simulink model "Expt2b"  (R2020b)
settings: Solver=VariableStepAuto  StartTime=0.0  StopTime=1.5  RelTol=1e-3
settings Model: Creator=geniu  LastModifiedBy=geniu

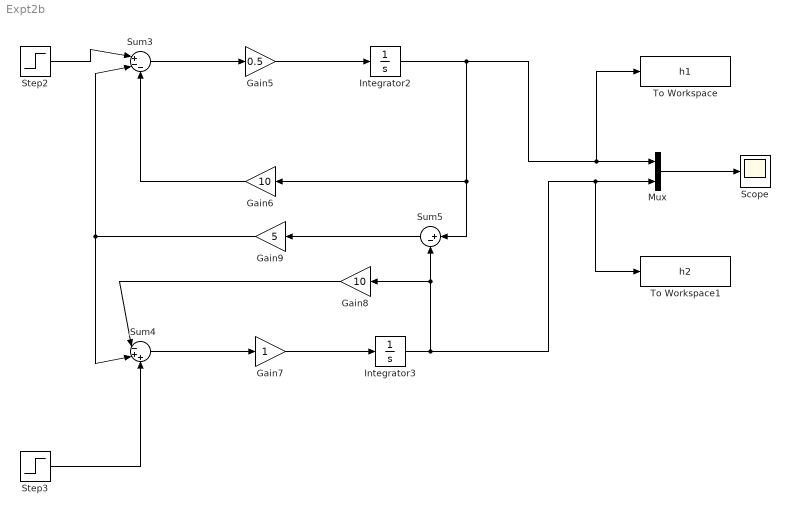
== system Expt2b ==
  Gain5 : Gain  Gain=0.5
  Gain6 : Gain  Gain=10
  Gain7 : Gain
  Gain8 : Gain  Gain=10
  Gain9 : Gain  Gain=5
  Integrator2 : Integrator
  Integrator3 : Integrator
  Mux : Mux  Inputs=2
  Scope : Scope
  Step2 : Step  Time=0  SampleTime=0
  Step3 : Step  Time=0  SampleTime=0
  Sum3 : Sum  Inputs=|+--
  Sum4 : Sum  Inputs=|-++
  Sum5 : Sum  Inputs=|+-
  To Workspace : ToWorkspace  VariableName=h1  SaveFormat=Timeseries  SampleTime=-1
  To Workspace1 : ToWorkspace  VariableName=h2  SaveFormat=Timeseries  SampleTime=-1
  wires:
  Gain9/1 -> Sum3/2, Sum4/2
  Sum5/1 -> Gain9/1
  Gain5/1 -> Integrator2/1
  Sum3/1 -> Gain5/1
  Gain7/1 -> Integrator3/1
  Step2/1 -> Sum3/1
  Step3/1 -> Sum4/3
  Gain8/1 -> Sum4/1
  Sum4/1 -> Gain7/1
  Integrator2/1 -> Gain6/1, Sum5/1, To Workspace/1, Mux/1
  Gain6/1 -> Sum3/3
  Integrator3/1 -> Gain8/1, Sum5/2, To Workspace1/1, Mux/2
  Mux/1 -> Scope/1
